simulink library "Lib_AC_PID"  (R2014b)
settings: Solver=ode45  StartTime=0.0  StopTime=10.0  RelTol=1e-3
undefined symbols (not defined in the file or in its folder): M_PI
libraries: Lib_AC_PID x8
settings Model: Creator=Ehang  LastModifiedBy=Ehang

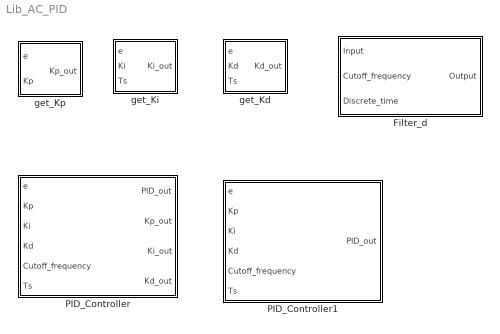
== system Lib_AC_PID ==
  Filter_d : Subsystem  Description=Tz是时间常数。时间常数一般不小于0.01，否则会振荡。
  PID_Controller : Subsystem  Description=PI控制器。
  PID_Controller1 : Subsystem  Description=PI控制器。
  get_Kd : Subsystem
  get_Ki : Subsystem
  get_Kp : Subsystem

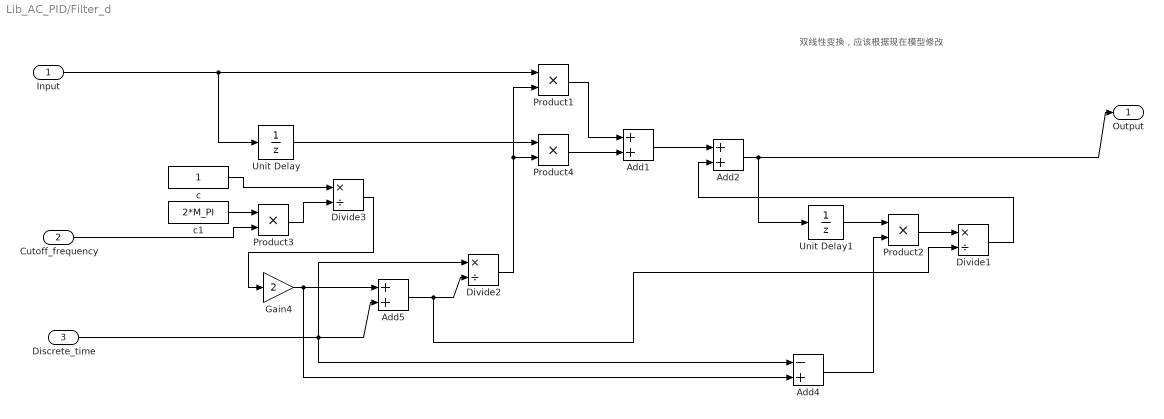
== system Lib_AC_PID/Filter_d ==
  note: 双线性变换，应该根据现在模型修改
  Input : Inport
  Cutoff_frequency : Inport  Port=2
  Discrete_time : Inport  Port=3
  Add1 : Sum
  Add2 : Sum
  Add4 : Sum  Inputs=-+
  Add5 : Sum
  Divide1 : Product  Inputs=*/
  Divide2 : Product  Inputs=*/
  Divide3 : Product  Inputs=*/
  Gain4 : Gain  Gain=2
  Product{1..4} (4 alike) : Product  RndMeth=Zero
  Unit Delay : UnitDelay  SampleTime=-1
  Unit Delay1 : UnitDelay  SampleTime=-1
  c : Constant  Description=低通滤波器的时间常数
  c1 : Constant  Description=低通滤波器的时间常数  Value=2*M_PI
  Output : Outport
  wires:
  Input/1 -> Unit Delay/1, Product1/1
  Add1/1 -> Add2/1
  Add2/1 -> Unit Delay1/1, Output/1
  Unit Delay1/1 -> Product2/1
  Gain4/1 -> Add5/1, Add4/2
  Discrete_time/1 -> Add4/1, Add5/2, Divide2/1
  Add5/1 -> Divide2/2, Divide1/2
  Add4/1 -> Product2/2
  Product2/1 -> Divide1/1
  Divide1/1 -> Add2/2
  Product1/1 -> Add1/1
  Divide2/1 -> Product1/2, Product4/2
  Product4/1 -> Add1/2
  Unit Delay/1 -> Product4/1
  c1/1 -> Product3/1
  Cutoff_frequency/1 -> Product3/2
  Product3/1 -> Divide3/2
  c/1 -> Divide3/1
  Divide3/1 -> Gain4/1

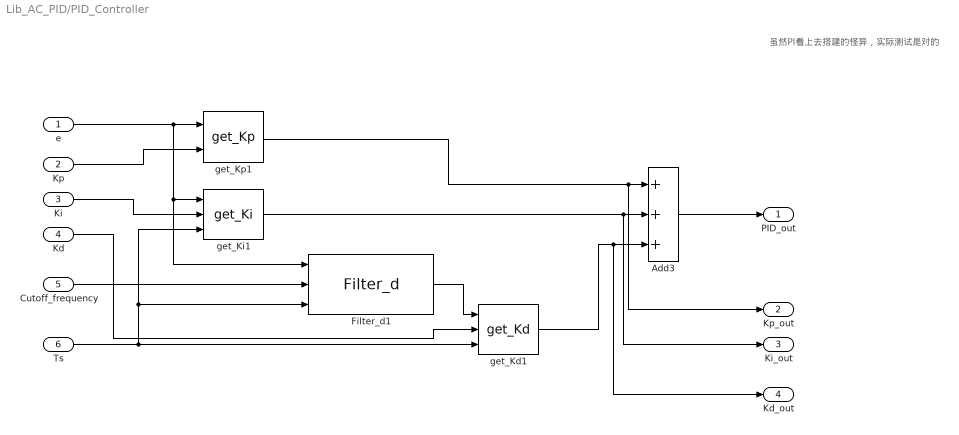
== system Lib_AC_PID/PID_Controller ==
  note: 虽然PI看上去搭建的怪异，实际测试是对的
  e : Inport
  Kp : Inport  Port=2
  Ki : Inport  Port=3
  Kd : Inport  Port=4
  Cutoff_frequency : Inport  Port=5
  Ts : Inport  Port=6
  Add3 : Sum  Inputs=+++
  Filter_d1 : Lib_AC_PID/Filter_d  Description=Tz是时间常数。时间常数一般不小于0.01，否则会振荡。
  get_Kd1 : Lib_AC_PID/get_Kd
  get_Ki1 : Lib_AC_PID/get_Ki
  get_Kp1 : Lib_AC_PID/get_Kp
  PID_out : Outport
  Kp_out : Outport  Port=2
  Ki_out : Outport  Port=3
  Kd_out : Outport  Port=4
  wires:
  get_Kp1/1 -> Kp_out/1, Add3/1
  get_Ki1/1 -> Ki_out/1, Add3/2
  get_Kd1/1 -> Kd_out/1, Add3/3
  Cutoff_frequency/1 -> Filter_d1/2
  Filter_d1/1 -> get_Kd1/1
  Kd/1 -> get_Kd1/2
  Ts/1 -> get_Kd1/3, Filter_d1/3, get_Ki1/3
  Ki/1 -> get_Ki1/2
  Kp/1 -> get_Kp1/2
  e/1 -> get_Kp1/1, Filter_d1/1, get_Ki1/1
  Add3/1 -> PID_out/1

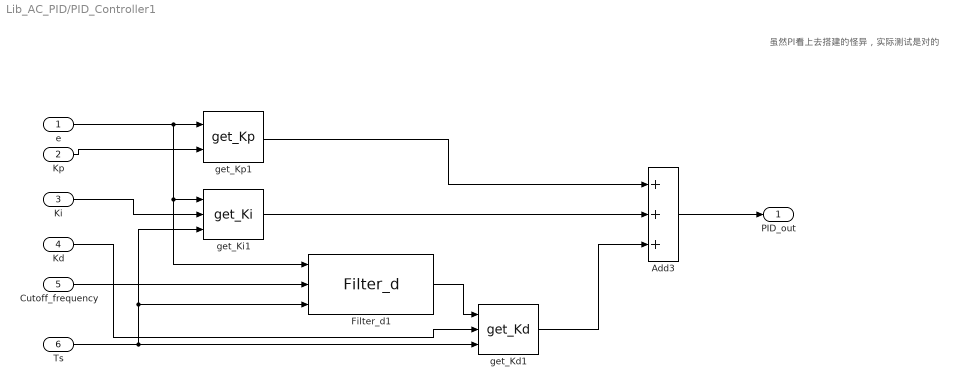
== system Lib_AC_PID/PID_Controller1 ==
  note: 虽然PI看上去搭建的怪异，实际测试是对的
  e : Inport
  Kp : Inport  Port=2
  Ki : Inport  Port=3
  Kd : Inport  Port=4
  Cutoff_frequency : Inport  Port=5
  Ts : Inport  Port=6
  Add3 : Sum  Inputs=+++
  Filter_d1 : Lib_AC_PID/Filter_d  Description=Tz是时间常数。时间常数一般不小于0.01，否则会振荡。
  get_Kd1 : Lib_AC_PID/get_Kd
  get_Ki1 : Lib_AC_PID/get_Ki
  get_Kp1 : Lib_AC_PID/get_Kp
  PID_out : Outport
  wires:
  Add3/1 -> PID_out/1
  e/1 -> get_Kp1/1, Filter_d1/1, get_Ki1/1
  Kp/1 -> get_Kp1/2
  Ki/1 -> get_Ki1/2
  Ts/1 -> get_Kd1/3, Filter_d1/3, get_Ki1/3
  Kd/1 -> get_Kd1/2
  Filter_d1/1 -> get_Kd1/1
  Cutoff_frequency/1 -> Filter_d1/2
  get_Kd1/1 -> Add3/3
  get_Ki1/1 -> Add3/2
  get_Kp1/1 -> Add3/1

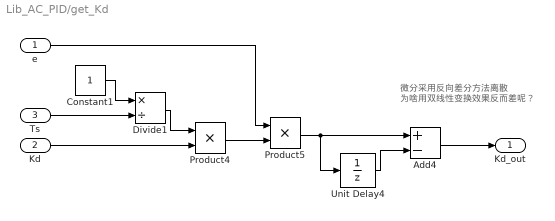
== system Lib_AC_PID/get_Kd ==
  note: 微分采用反向差分方法离散
      | 为啥用双线性变换效果反而差呢？
  e : Inport
  Kd : Inport  Port=2
  Ts : Inport  Port=3
  Add4 : Sum  Inputs=+-
  Constant1 : Constant
  Divide1 : Product  Inputs=*/
  Product4 : Product  RndMeth=Zero
  Product5 : Product  RndMeth=Zero
  Unit Delay4 : UnitDelay  SampleTime=-1
  Kd_out : Outport
  wires:
  Product4/1 -> Product5/2
  Product5/1 -> Add4/1, Unit Delay4/1
  Constant1/1 -> Divide1/1
  Divide1/1 -> Product4/1
  Unit Delay4/1 -> Add4/2
  Ts/1 -> Divide1/2
  e/1 -> Product5/1
  Add4/1 -> Kd_out/1
  Kd/1 -> Product4/2

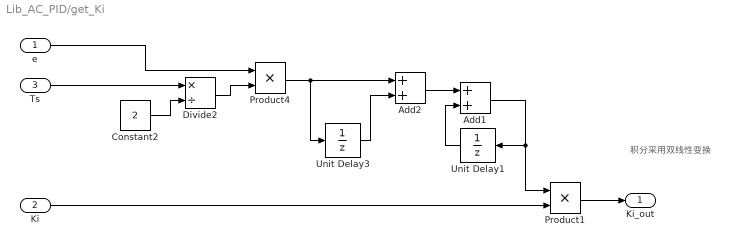
== system Lib_AC_PID/get_Ki ==
  note: 积分采用双线性变换
  e : Inport
  Ki : Inport  Port=2
  Ts : Inport  Port=3
  Add1 : Sum
  Add2 : Sum
  Constant2 : Constant  Value=2
  Divide2 : Product  Inputs=*/
  Product1 : Product  RndMeth=Zero
  Product4 : Product  RndMeth=Zero
  Unit Delay1 : UnitDelay  SampleTime=-1
  Unit Delay3 : UnitDelay  SampleTime=-1
  Ki_out : Outport
  wires:
  Add2/1 -> Add1/1
  Unit Delay1/1 -> Add1/2
  Ts/1 -> Divide2/1
  Constant2/1 -> Divide2/2
  Add1/1 -> Unit Delay1/1, Product1/1
  Ki/1 -> Product1/2
  Product1/1 -> Ki_out/1
  Divide2/1 -> Product4/2
  e/1 -> Product4/1
  Product4/1 -> Add2/1, Unit Delay3/1
  Unit Delay3/1 -> Add2/2

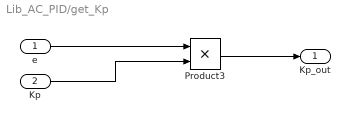
== system Lib_AC_PID/get_Kp ==
  e : Inport
  Kp : Inport  Port=2
  Product3 : Product  RndMeth=Zero
  Kp_out : Outport
  wires:
  Kp/1 -> Product3/2
  Product3/1 -> Kp_out/1
  e/1 -> Product3/1
